simulink model "PulseCodeModulation"  (R2017a)
settings: Solver=VariableStepAuto  StartTime=0.0  StopTime=.5  RelTol=1e-3
libraries: commutil2 x2, commsrccod2 x2
settings Model: Creator=j  LastModifiedBy=j

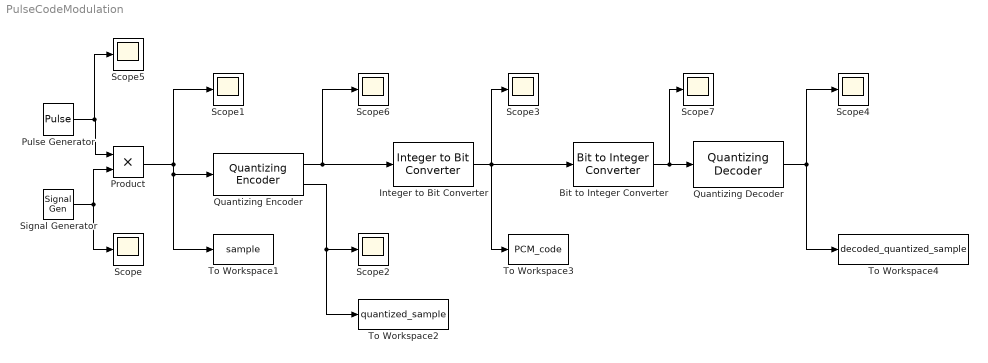
== system PulseCodeModulation ==
  Bit to Integer Converter : commutil2/Bit to Integer Converter  nbits=2  bitOrder=MSB first  signedOutputValues=Unsigned  outDtype=Inherit via internal rule  outDtypeSigned=Inherit via internal rule
  Integer to Bit Converter : commutil2/Integer to Bit Converter  nbits=2  signedInputValues=Unsigned  bitOrder=MSB first  outDtype=Inherit via internal rule
  Product : Product
  Pulse Generator : DiscretePulseGenerator  PulseType=Time based  Period=0.01
  Quantizing Decoder : commsrccod2/Quantizing Decoder  codebook=[-.75 -.25 .25 .75]  QuDType=double
      settings: SourceProductName=Communications System Toolbox  SourceProductBaseCode=CM
  Quantizing Encoder : commsrccod2/Quantizing Encoder  partition=[-.5 0 .5]  codebook=[-.75 -.25 .25 .75]  idxDType=double
      settings: SourceProductName=Communications System Toolbox  SourceProductBaseCode=CM
  Scope{,1..7} (8 alike) : Scope
  Signal Generator : SignalGenerator  Frequency=5
  To Workspace1 : ToWorkspace  VariableName=sample  SampleTime=0.01
  To Workspace2 : ToWorkspace  VariableName=quantized_sample  SampleTime=0.01
  To Workspace3 : ToWorkspace  VariableName=PCM_code  SampleTime=0.01
  To Workspace4 : ToWorkspace  VariableName=decoded_quantized_sample  SampleTime=0.01
  wires:
  Pulse Generator/1 -> Scope5/1, Product/1
  Signal Generator/1 -> Scope/1, Product/2
  Product/1 -> Quantizing Encoder/1, To Workspace1/1, Scope1/1
  Integer to Bit Converter/1 -> To Workspace3/1, Bit to Integer Converter/1, Scope3/1
  Quantizing Decoder/1 -> To Workspace4/1, Scope4/1
  Quantizing Encoder/1 -> Scope6/1, Integer to Bit Converter/1
  Quantizing Encoder/2 -> To Workspace2/1, Scope2/1
  Bit to Integer Converter/1 -> Scope7/1, Quantizing Decoder/1
